simulink library "VIS_LIB"  (Simulink 8.6)
settings: Solver=ode45  StartTime=0.0  StopTime=10.0  RelTol=1e-3
undefined symbols (not defined in the file): AC, SIXOSEM_F_WD_AC_MASTER
libraries: cdsFilt x376, cdsEpicsOut x253, cdsEpicsIn x179, cdsTP x123, VIS_LIB x95, cdsMuxMatrix x91, cdsEpicsStringIn x75, cdsFiltCtrl x72, cdsFunctionCall x70, cdsRms x59, KAGRA_UTIL x25, STATE_BIO_MASTER x5
(part 29 of 38)

== system VIS_LIB/MODAL/inputproc/CAL_GAS ==
  note: #DAQ Channels
      |
      | M1_OUT 256
      | M2_OUT 256
      | M3_OUT 256
      | M4_OUT 256
      | M5_OUT 256
      | M1_IN1 128
      | M2_IN1 128
      | M3_IN1 128
      | M4_IN1 128
      | M5_IN1 128
  LEN_IN : Inport
  TRA_IN : Inport  Port=2
  VER_IN : Inport  Port=3
  ROL_IN : Inport  Port=4
  PIT_IN : Inport  Port=5
  M1 : cdsFilt/Subsystem  Tag=cdsFilt  Description=|
      | Purpose:                                                                                                                                                                                                                                  
      | Standard CDS IIR filter module.                                                                                                                                                                                                           
      |                                                                                                                                                                                                                                           
      | Operation:                                                                                                                                                                                                                                
      | Consists of 10 second order section IIR filters, plus a ramped gain stage. In FE code, also provides pre-defined test points and excitation channel inputs. The filter coefficients are defined in the LIGO system using the 'foton' tool.
      |                                                                                                                                                                                                                                           
      | Usage:                                                                                                                                                                                                                                    
      | Name the part with the desired filter module name.
      settings: AttributesFormatString=%<Tag>
  M2 : cdsFilt/Subsystem  Tag=cdsFilt  Description=|
      | Purpose:                                                                                                                                                                                                                                  
      | Standard CDS IIR filter module.                                                                                                                                                                                                           
      |                                                                                                                                                                                                                                           
      | Operation:                                                                                                                                                                                                                                
      | Consists of 10 second order section IIR filters, plus a ramped gain stage. In FE code, also provides pre-defined test points and excitation channel inputs. The filter coefficients are defined in the LIGO system using the 'foton' tool.
      |                                                                                                                                                                                                                                           
      | Usage:                                                                                                                                                                                                                                    
      | Name the part with the desired filter module name.
      settings: AttributesFormatString=%<Tag>
  M3 : cdsFilt/Subsystem  Tag=cdsFilt  Description=|
      | Purpose:                                                                                                                                                                                                                                  
      | Standard CDS IIR filter module.                                                                                                                                                                                                           
      |                                                                                                                                                                                                                                           
      | Operation:                                                                                                                                                                                                                                
      | Consists of 10 second order section IIR filters, plus a ramped gain stage. In FE code, also provides pre-defined test points and excitation channel inputs. The filter coefficients are defined in the LIGO system using the 'foton' tool.
      |                                                                                                                                                                                                                                           
      | Usage:                                                                                                                                                                                                                                    
      | Name the part with the desired filter module name.
      settings: AttributesFormatString=%<Tag>
  M4 : cdsFilt/Subsystem  Tag=cdsFilt  Description=|
      | Purpose:                                                                                                                                                                                                                                  
      | Standard CDS IIR filter module.                                                                                                                                                                                                           
      |                                                                                                                                                                                                                                           
      | Operation:                                                                                                                                                                                                                                
      | Consists of 10 second order section IIR filters, plus a ramped gain stage. In FE code, also provides pre-defined test points and excitation channel inputs. The filter coefficients are defined in the LIGO system using the 'foton' tool.
      |                                                                                                                                                                                                                                           
      | Usage:                                                                                                                                                                                                                                    
      | Name the part with the desired filter module name.
      settings: AttributesFormatString=%<Tag>
  M5 : cdsFilt/Subsystem  Tag=cdsFilt  Description=|
      | Purpose:                                                                                                                                                                                                                                  
      | Standard CDS IIR filter module.                                                                                                                                                                                                           
      |                                                                                                                                                                                                                                           
      | Operation:                                                                                                                                                                                                                                
      | Consists of 10 second order section IIR filters, plus a ramped gain stage. In FE code, also provides pre-defined test points and excitation channel inputs. The filter coefficients are defined in the LIGO system using the 'foton' tool.
      |                                                                                                                                                                                                                                           
      | Usage:                                                                                                                                                                                                                                    
      | Name the part with the desired filter module name.
      settings: AttributesFormatString=%<Tag>
  LEN_OUT : Outport
  TRA_OUT : Outport  Port=2
  VER_OUT : Outport  Port=3
  ROL_OUT : Outport  Port=4
  PIT_OUT : Outport  Port=5
  wires:
  M1/1 -> LEN_OUT/1
  LEN_IN/1 -> M1/1
  M5/1 -> PIT_OUT/1
  PIT_IN/1 -> M5/1
  ROL_IN/1 -> M4/1
  M4/1 -> ROL_OUT/1
  M2/1 -> TRA_OUT/1
  TRA_IN/1 -> M2/1
  VER_IN/1 -> M3/1
  M3/1 -> VER_OUT/1

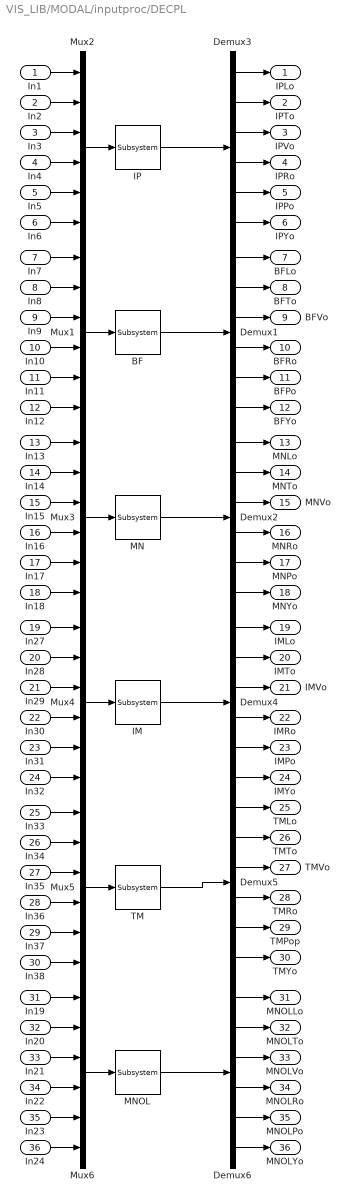
== system VIS_LIB/MODAL/inputproc/DECPL ==
  In1 : Inport
  In2 : Inport  Port=2
  In3 : Inport  Port=3
  In4 : Inport  Port=4
  In5 : Inport  Port=5
  In6 : Inport  Port=6
  In7 : Inport  Port=7
  In8 : Inport  Port=8
  In9 : Inport  Port=9
  In10 : Inport  Port=10
  In11 : Inport  Port=11
  In12 : Inport  Port=12
  In13 : Inport  Port=13
  In14 : Inport  Port=14
  In15 : Inport  Port=15
  In16 : Inport  Port=16
  In17 : Inport  Port=17
  In18 : Inport  Port=18
  In27 : Inport  Port=19
  In28 : Inport  Port=20
  In29 : Inport  Port=21
  In30 : Inport  Port=22
  In31 : Inport  Port=23
  In32 : Inport  Port=24
  In33 : Inport  Port=25
  In34 : Inport  Port=26
  In35 : Inport  Port=27
  In36 : Inport  Port=28
  In37 : Inport  Port=29
  In38 : Inport  Port=30
  In19 : Inport  Port=31
  In20 : Inport  Port=32
  In21 : Inport  Port=33
  In22 : Inport  Port=34
  In23 : Inport  Port=35
  In24 : Inport  Port=36
  BF : cdsMuxMatrix/Subsystem  Tag=cdsMuxMatrix  Description=Any size matrix. Inputs and outputs must be connected using Mux and Demux parts.
      settings: AttributesFormatString=%<Tag>
  Demux{1..6} (6 alike) : Demux  Outputs=6
  IM : cdsMuxMatrix/Subsystem  Tag=cdsMuxMatrix  Description=Any size matrix. Inputs and outputs must be connected using Mux and Demux parts.
      settings: AttributesFormatString=%<Tag>
  IP : cdsMuxMatrix/Subsystem  Tag=cdsMuxMatrix  Description=Any size matrix. Inputs and outputs must be connected using Mux and Demux parts.
      settings: AttributesFormatString=%<Tag>
  MN : cdsMuxMatrix/Subsystem  Tag=cdsMuxMatrix  Description=Any size matrix. Inputs and outputs must be connected using Mux and Demux parts.
      settings: AttributesFormatString=%<Tag>
  MNOL : cdsMuxMatrix/Subsystem  Tag=cdsMuxMatrix  Description=Any size matrix. Inputs and outputs must be connected using Mux and Demux parts.
      settings: AttributesFormatString=%<Tag>
  Mux{1..6} (6 alike) : Mux  Inputs=6
  TM : cdsMuxMatrix/Subsystem  Tag=cdsMuxMatrix  Description=Any size matrix. Inputs and outputs must be connected using Mux and Demux parts.
      settings: AttributesFormatString=%<Tag>
  IPLo : Outport
  IPTo : Outport  Port=2
  IPVo : Outport  Port=3
  IPRo : Outport  Port=4
  IPPo : Outport  Port=5
  IPYo : Outport  Port=6
  BFLo : Outport  Port=7
  BFTo : Outport  Port=8
  BFVo : Outport  Port=9
  BFRo : Outport  Port=10
  BFPo : Outport  Port=11
  BFYo : Outport  Port=12
  MNLo : Outport  Port=13
  MNTo : Outport  Port=14
  MNVo : Outport  Port=15
  MNRo : Outport  Port=16
  MNPo : Outport  Port=17
  MNYo : Outport  Port=18
  IMLo : Outport  Port=19
  IMTo : Outport  Port=20
  IMVo : Outport  Port=21
  IMRo : Outport  Port=22
  IMPo : Outport  Port=23
  IMYo : Outport  Port=24
  TMLo : Outport  Port=25
  TMTo : Outport  Port=26
  TMVo : Outport  Port=27
  TMRo : Outport  Port=28
  TMPop : Outport  Port=29
  TMYo : Outport  Port=30
  MNOLLo : Outport  Port=31
  MNOLTo : Outport  Port=32
  MNOLVo : Outport  Port=33
  MNOLRo : Outport  Port=34
  MNOLPo : Outport  Port=35
  MNOLYo : Outport  Port=36
  wires:
  In6/1 -> Mux2/6
  Mux2/1 -> IP/1
  In3/1 -> Mux2/3
  In1/1 -> Mux2/1
  IP/1 -> Demux3/1
  In5/1 -> Mux2/5
  In2/1 -> Mux2/2
  In4/1 -> Mux2/4
  In12/1 -> Mux1/6
  Mux1/1 -> BF/1
  In9/1 -> Mux1/3
  In7/1 -> Mux1/1
  BF/1 -> Demux1/1
  In11/1 -> Mux1/5
  In8/1 -> Mux1/2
  In10/1 -> Mux1/4
  In18/1 -> Mux3/6
  Mux3/1 -> MN/1
  In15/1 -> Mux3/3
  In13/1 -> Mux3/1
  MN/1 -> Demux2/1
  In17/1 -> Mux3/5
  In14/1 -> Mux3/2
  In16/1 -> Mux3/4
  Mux4/1 -> IM/1
  IM/1 -> Demux4/1
  In30/1 -> Mux4/4
  In27/1 -> Mux4/1
  In29/1 -> Mux4/3
  In28/1 -> Mux4/2
  In32/1 -> Mux4/6
  In31/1 -> Mux4/5
  In38/1 -> Mux5/6
  Mux5/1 -> TM/1
  In35/1 -> Mux5/3
  In33/1 -> Mux5/1
  TM/1 -> Demux5/1
  In37/1 -> Mux5/5
  In34/1 -> Mux5/2
  In36/1 -> Mux5/4
  Demux3/6 -> IPYo/1
  Demux1/1 -> BFLo/1
  Demux1/2 -> BFTo/1
  Demux1/3 -> BFVo/1
  Demux1/4 -> BFRo/1
  Demux1/5 -> BFPo/1
  Demux1/6 -> BFYo/1
  Demux2/1 -> MNLo/1
  Demux2/2 -> MNTo/1
  Demux2/3 -> MNVo/1
  Demux2/4 -> MNRo/1
  Demux2/5 -> MNPo/1
  Demux2/6 -> MNYo/1
  Demux4/1 -> IMLo/1
  Demux4/2 -> IMTo/1
  Demux4/3 -> IMVo/1
  Demux4/4 -> IMRo/1
  Demux4/5 -> IMPo/1
  Demux4/6 -> IMYo/1
  Demux5/1 -> TMLo/1
  Demux3/1 -> IPLo/1
  Demux3/2 -> IPTo/1
  Demux3/3 -> IPVo/1
  Demux3/4 -> IPRo/1
  Demux3/5 -> IPPo/1
  Demux5/2 -> TMTo/1
  Demux5/3 -> TMVo/1
  Demux5/4 -> TMRo/1
  Demux5/5 -> TMPop/1
  Demux5/6 -> TMYo/1
  In24/1 -> Mux6/6
  Mux6/1 -> MNOL/1
  In21/1 -> Mux6/3
  In19/1 -> Mux6/1
  MNOL/1 -> Demux6/1
  In23/1 -> Mux6/5
  In20/1 -> Mux6/2
  In22/1 -> Mux6/4
  Demux6/2 -> MNOLTo/1
  Demux6/3 -> MNOLVo/1
  Demux6/4 -> MNOLRo/1
  Demux6/5 -> MNOLPo/1
  Demux6/6 -> MNOLYo/1
  Demux6/1 -> MNOLLo/1

== system VIS_LIB/MODAL/inputproc/EUL ==
  In1 : Inport
  In2 : Inport  Port=2
  In3 : Inport  Port=3
  In4 : Inport  Port=4
  In5 : Inport  Port=5
  In6 : Inport  Port=6
  In7 : Inport  Port=7
  In8 : Inport  Port=8
  In9 : Inport  Port=9
  In10 : Inport  Port=10
  In11 : Inport  Port=11
  In12 : Inport  Port=12
  In13 : Inport  Port=13
  In14 : Inport  Port=14
  In15 : Inport  Port=15
  In16 : Inport  Port=16
  In17 : Inport  Port=17
  In18 : Inport  Port=18
  In19 : Inport  Port=19
  In20 : Inport  Port=20
  In21 : Inport  Port=21
  In22 : Inport  Port=22
  In23 : Inport  Port=23
  In24 : Inport  Port=24
  In25 : Inport  Port=25
  In26 : Inport  Port=26
  In27 : Inport  Port=27
  In28 : Inport  Port=28
  In29 : Inport  Port=29
  In30 : Inport  Port=30
  In31 : Inport  Port=31
  In32 : Inport  Port=32
  In33 : Inport  Port=33
  In34 : Inport  Port=34
  In35 : Inport  Port=35
  In36 : Inport  Port=36
  BF : VIS_LIB/UTILs/FBs_6DOF_DQ
  IM : VIS_LIB/UTILs/FBs_6DOF_DQ
  IP : VIS_LIB/UTILs/FBs_6DOF_DQ
  MN : VIS_LIB/UTILs/FBs_6DOF_DQ
  MNOL : VIS_LIB/UTILs/FBs_6DOF_DQ
  TM : VIS_LIB/UTILs/FBs_6DOF_DQ
  Out1 : Outport
  Out2 : Outport  Port=2
  Out3 : Outport  Port=3
  Out4 : Outport  Port=4
  Out5 : Outport  Port=5
  Out6 : Outport  Port=6
  Out7 : Outport  Port=7
  Out8 : Outport  Port=8
  Out9 : Outport  Port=9
  Out10 : Outport  Port=10
  Out11 : Outport  Port=11
  Out12 : Outport  Port=12
  Out13 : Outport  Port=13
  Out14 : Outport  Port=14
  Out15 : Outport  Port=15
  Out16 : Outport  Port=16
  Out17 : Outport  Port=17
  Out18 : Outport  Port=18
  Out19 : Outport  Port=19
  Out20 : Outport  Port=20
  Out21 : Outport  Port=21
  Out22 : Outport  Port=22
  Out23 : Outport  Port=23
  Out24 : Outport  Port=24
  Out25 : Outport  Port=25
  Out26 : Outport  Port=26
  Out27 : Outport  Port=27
  Out28 : Outport  Port=28
  Out29 : Outport  Port=29
  Out30 : Outport  Port=30
  Out31 : Outport  Port=31
  Out32 : Outport  Port=32
  Out33 : Outport  Port=33
  Out34 : Outport  Port=34
  Out35 : Outport  Port=35
  Out36 : Outport  Port=36
  wires:
  In16/1 -> MN/4
  In15/1 -> MN/3
  In14/1 -> MN/2
  In12/1 -> BF/6
  In13/1 -> MN/1
  In11/1 -> BF/5
  In10/1 -> BF/4
  In9/1 -> BF/3
  In8/1 -> BF/2
  TM/5 -> Out29/1
  TM/2 -> Out26/1
  TM/3 -> Out27/1
  In30/1 -> TM/6
  TM/1 -> Out25/1
  In23/1 -> IM/5
  In22/1 -> IM/4
  In21/1 -> IM/3
  In20/1 -> IM/2
  BF/6 -> Out12/1
  In19/1 -> IM/1
  MN/2 -> Out14/1
  MN/1 -> Out13/1
  In17/1 -> MN/5
  In18/1 -> MN/6
  IM/2 -> Out20/1
  MN/3 -> Out15/1
  IM/1 -> Out19/1
  In24/1 -> IM/6
  TM/4 -> Out28/1
  BF/1 -> Out7/1
  MN/6 -> Out18/1
  MN/5 -> Out17/1
  MN/4 -> Out16/1
  TM/6 -> Out30/1
  In7/1 -> BF/1
  In6/1 -> IP/6
  In5/1 -> IP/5
  In3/1 -> IP/3
  In4/1 -> IP/4
  In29/1 -> TM/5
  In28/1 -> TM/4
  In27/1 -> TM/3
  In26/1 -> TM/2
  BF/5 -> Out11/1
  BF/4 -> Out10/1
  BF/3 -> Out9/1
  BF/2 -> Out8/1
  IP/3 -> Out3/1
  IP/2 -> Out2/1
  IP/1 -> Out1/1
  In1/1 -> IP/1
  In25/1 -> TM/1
  IM/6 -> Out24/1
  IM/5 -> Out23/1
  IM/3 -> Out21/1
  IM/4 -> Out22/1
  In2/1 -> IP/2
  IP/6 -> Out6/1
  IP/5 -> Out5/1
  IP/4 -> Out4/1
  MNOL/5 -> Out35/1
  MNOL/2 -> Out32/1
  MNOL/3 -> Out33/1
  In36/1 -> MNOL/6
  MNOL/4 -> Out34/1
  MNOL/6 -> Out36/1
  In35/1 -> MNOL/5
  In34/1 -> MNOL/4
  In33/1 -> MNOL/3
  In32/1 -> MNOL/2
  In31/1 -> MNOL/1
  MNOL/1 -> Out31/1

== system VIS_LIB/MODAL/inputproc/OL_PROC ==
  MNSEG1 : Inport
  MNSEG2 : Inport  Port=2
  MNSEG3 : Inport  Port=3
  MNSEG4 : Inport  Port=4
  TILT_SEG1 : Inport  Port=5
  TILT_SEG2 : Inport  Port=6
  TILT_SEG3 : Inport  Port=7
  TILT_SEG4 : Inport  Port=8
  LEN_SEG1 : Inport  Port=9
  LEN_SEG2 : Inport  Port=10
  LEN_SEG3 : Inport  Port=11
  LEN_SEG4 : Inport  Port=12
  MN_TILT : Subsystem
  TM_LEN : Subsystem
  TM_TILT : Subsystem
  MNV : Outport
  MNH : Outport  Port=2
  TMV1 : Outport  Port=3
  TMV2 : Outport  Port=4
  TMH1 : Outport  Port=5
  TMH2 : Outport  Port=6
  wires:
  MNSEG2/1 -> MN_TILT/2(SEG2_in)
  MNSEG1/1 -> MN_TILT/1(SEG1_in)
  MNSEG4/1 -> MN_TILT/4(SEG4_in)
  MN_TILT/1(V) -> MNV/1
  MN_TILT/2(H) -> MNH/1
  MNSEG3/1 -> MN_TILT/3(SEG3_in)
  TILT_SEG1/1 -> TM_TILT/1(SEG1_in)
  TILT_SEG2/1 -> TM_TILT/2(SEG2_in)
  TILT_SEG4/1 -> TM_TILT/4(SEG4_in)
  TILT_SEG3/1 -> TM_TILT/3(SEG3_in)
  LEN_SEG1/1 -> TM_LEN/1(SEG1_in)
  LEN_SEG2/1 -> TM_LEN/2(SEG2_in)
  LEN_SEG3/1 -> TM_LEN/3(SEG3_in)
  LEN_SEG4/1 -> TM_LEN/4(SEG4_in)
  TM_TILT/1(V) -> TMV1/1
  TM_TILT/2(H) -> TMH1/1
  TM_LEN/1(V) -> TMV2/1
  TM_LEN/2(H) -> TMH2/1

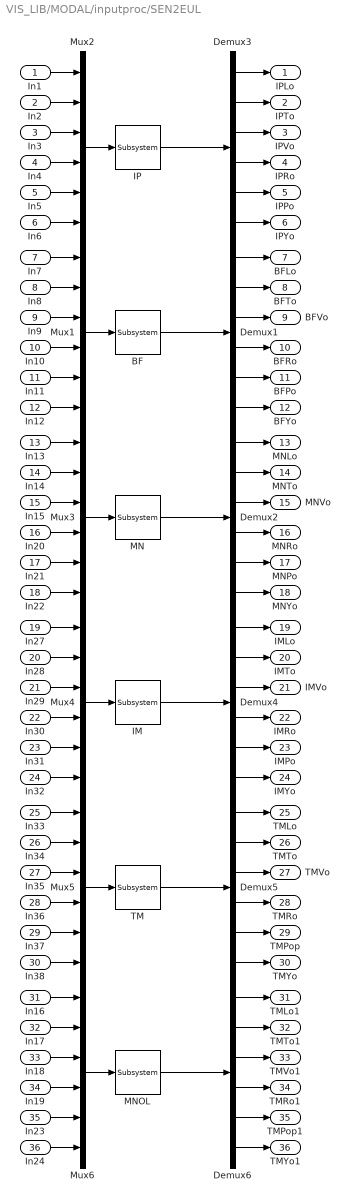
== system VIS_LIB/MODAL/inputproc/SEN2EUL ==
  In1 : Inport
  In2 : Inport  Port=2
  In3 : Inport  Port=3
  In4 : Inport  Port=4
  In5 : Inport  Port=5
  In6 : Inport  Port=6
  In7 : Inport  Port=7
  In8 : Inport  Port=8
  In9 : Inport  Port=9
  In10 : Inport  Port=10
  In11 : Inport  Port=11
  In12 : Inport  Port=12
  In13 : Inport  Port=13
  In14 : Inport  Port=14
  In15 : Inport  Port=15
  In20 : Inport  Port=16
  In21 : Inport  Port=17
  In22 : Inport  Port=18
  In27 : Inport  Port=19
  In28 : Inport  Port=20
  In29 : Inport  Port=21
  In30 : Inport  Port=22
  In31 : Inport  Port=23
  In32 : Inport  Port=24
  In33 : Inport  Port=25
  In34 : Inport  Port=26
  In35 : Inport  Port=27
  In36 : Inport  Port=28
  In37 : Inport  Port=29
  In38 : Inport  Port=30
  In16 : Inport  Port=31
  In17 : Inport  Port=32
  In18 : Inport  Port=33
  In19 : Inport  Port=34
  In23 : Inport  Port=35
  In24 : Inport  Port=36
  BF : cdsMuxMatrix/Subsystem  Tag=cdsMuxMatrix  Description=Any size matrix. Inputs and outputs must be connected using Mux and Demux parts.
      settings: AttributesFormatString=%<Tag>
  Demux{1..6} (6 alike) : Demux  Outputs=6
  IM : cdsMuxMatrix/Subsystem  Tag=cdsMuxMatrix  Description=Any size matrix. Inputs and outputs must be connected using Mux and Demux parts.
      settings: AttributesFormatString=%<Tag>
  IP : cdsMuxMatrix/Subsystem  Tag=cdsMuxMatrix  Description=Any size matrix. Inputs and outputs must be connected using Mux and Demux parts.
      settings: AttributesFormatString=%<Tag>
  MN : cdsMuxMatrix/Subsystem  Tag=cdsMuxMatrix  Description=Any size matrix. Inputs and outputs must be connected using Mux and Demux parts.
      settings: AttributesFormatString=%<Tag>
  MNOL : cdsMuxMatrix/Subsystem  Tag=cdsMuxMatrix  Description=Any size matrix. Inputs and outputs must be connected using Mux and Demux parts.
      settings: AttributesFormatString=%<Tag>
  Mux{1..6} (6 alike) : Mux  Inputs=6
  TM : cdsMuxMatrix/Subsystem  Tag=cdsMuxMatrix  Description=Any size matrix. Inputs and outputs must be connected using Mux and Demux parts.
      settings: AttributesFormatString=%<Tag>
  IPLo : Outport
  IPTo : Outport  Port=2
  IPVo : Outport  Port=3
  IPRo : Outport  Port=4
  IPPo : Outport  Port=5
  IPYo : Outport  Port=6
  BFLo : Outport  Port=7
  BFTo : Outport  Port=8
  BFVo : Outport  Port=9
  BFRo : Outport  Port=10
  BFPo : Outport  Port=11
  BFYo : Outport  Port=12
  MNLo : Outport  Port=13
  MNTo : Outport  Port=14
  MNVo : Outport  Port=15
  MNRo : Outport  Port=16
  MNPo : Outport  Port=17
  MNYo : Outport  Port=18
  IMLo : Outport  Port=19
  IMTo : Outport  Port=20
  IMVo : Outport  Port=21
  IMRo : Outport  Port=22
  IMPo : Outport  Port=23
  IMYo : Outport  Port=24
  TMLo : Outport  Port=25
  TMTo : Outport  Port=26
  TMVo : Outport  Port=27
  TMRo : Outport  Port=28
  TMPop : Outport  Port=29
  TMYo : Outport  Port=30
  TMLo1 : Outport  Port=31
  TMTo1 : Outport  Port=32
  TMVo1 : Outport  Port=33
  TMRo1 : Outport  Port=34
  TMPop1 : Outport  Port=35
  TMYo1 : Outport  Port=36
  wires:
  In6/1 -> Mux2/6
  Mux2/1 -> IP/1
  In3/1 -> Mux2/3
  In1/1 -> Mux2/1
  IP/1 -> Demux3/1
  In5/1 -> Mux2/5
  In2/1 -> Mux2/2
  In4/1 -> Mux2/4
  In12/1 -> Mux1/6
  Mux1/1 -> BF/1
  In9/1 -> Mux1/3
  In7/1 -> Mux1/1
  BF/1 -> Demux1/1
  In11/1 -> Mux1/5
  In8/1 -> Mux1/2
  In10/1 -> Mux1/4
  Mux3/1 -> MN/1
  In15/1 -> Mux3/3
  In13/1 -> Mux3/1
  MN/1 -> Demux2/1
  In14/1 -> Mux3/2
  Mux4/1 -> IM/1
  IM/1 -> Demux4/1
  In21/1 -> Mux3/5
  In20/1 -> Mux3/4
  In22/1 -> Mux3/6
  In30/1 -> Mux4/4
  In27/1 -> Mux4/1
  In29/1 -> Mux4/3
  In28/1 -> Mux4/2
  In32/1 -> Mux4/6
  In31/1 -> Mux4/5
  In38/1 -> Mux5/6
  Mux5/1 -> TM/1
  In35/1 -> Mux5/3
  In33/1 -> Mux5/1
  TM/1 -> Demux5/1
  In37/1 -> Mux5/5
  In34/1 -> Mux5/2
  In36/1 -> Mux5/4
  Demux3/6 -> IPYo/1
  Demux1/1 -> BFLo/1
  Demux1/2 -> BFTo/1
  Demux1/3 -> BFVo/1
  Demux1/4 -> BFRo/1
  Demux1/5 -> BFPo/1
  Demux1/6 -> BFYo/1
  Demux2/1 -> MNLo/1
  Demux2/2 -> MNTo/1
  Demux2/3 -> MNVo/1
  Demux2/4 -> MNRo/1
  Demux2/5 -> MNPo/1
  Demux2/6 -> MNYo/1
  Demux4/1 -> IMLo/1
  Demux4/2 -> IMTo/1
  Demux4/3 -> IMVo/1
  Demux4/4 -> IMRo/1
  Demux4/5 -> IMPo/1
  Demux4/6 -> IMYo/1
  Demux5/1 -> TMLo/1
  Demux3/1 -> IPLo/1
  Demux3/2 -> IPTo/1
  Demux3/3 -> IPVo/1
  Demux3/4 -> IPRo/1
  Demux3/5 -> IPPo/1
  Demux5/2 -> TMTo/1
  Demux5/3 -> TMVo/1
  Demux5/4 -> TMRo/1
  Demux5/5 -> TMPop/1
  Demux5/6 -> TMYo/1
  In24/1 -> Mux6/6
  Mux6/1 -> MNOL/1
  In18/1 -> Mux6/3
  MNOL/1 -> Demux6/1
  In23/1 -> Mux6/5
  In17/1 -> Mux6/2
  In19/1 -> Mux6/4
  Demux6/2 -> TMTo1/1
  Demux6/3 -> TMVo1/1
  Demux6/4 -> TMRo1/1
  Demux6/5 -> TMPop1/1
  Demux6/6 -> TMYo1/1
  Demux6/1 -> TMLo1/1
  In16/1 -> Mux6/1

== system VIS_LIB/MODAL/inputproc/SENSIN ==
  IPLVDT_H1 : Inport
  IPLVDT_H2 : Inport  Port=2
  IPLVDT_H3 : Inport  Port=3
  BFLVDT_V1 : Inport  Port=4
  BFLVDT_V2 : Inport  Port=5
  BFLVDT_V3 : Inport  Port=6
  BFLVDT_H1 : Inport  Port=7
  BFLVDT_H2 : Inport  Port=8
  BFLVDT_H3 : Inport  Port=9
  MCPS_V1 : Inport  Port=10
  MCPS_V2 : Inport  Port=11
  MCPS_V3 : Inport  Port=12
  MCPS_H1 : Inport  Port=13
  MCPS_H2 : Inport  Port=14
  MNPS_H3 : Inport  Port=15
  IMPS_V1 : Inport  Port=16
  IMPS_V2 : Inport  Port=17
  IMPS_V3 : Inport  Port=18
  IMPS_H1 : Inport  Port=19
  IMPS_H2 : Inport  Port=20
  IMPS_H3 : Inport  Port=21
  MNOL_V : Inport  Port=22
  MNOL_H4 : Inport  Port=23
  TMOLV1 : Inport  Port=24
  TMOLV2 : Inport  Port=25
  TMOLH1 : Inport  Port=26
  TMOLH2 : Inport  Port=27
  BF : VIS_LIB/UTILs/6COILs_DQ
  Ground{1..7,9..10} (9 alike) : Ground
  IM : VIS_LIB/UTILs/6COILs_DQ
  IP : VIS_LIB/UTILs/6COILs_DQ
  MN : VIS_LIB/UTILs/6COILs_DQ
  MNOL : VIS_LIB/UTILs/6COILs_DQ
  TM : VIS_LIB/UTILs/6COILs_DQ
  IPV1 : Outport
  IPV2 : Outport  Port=2
  IPV3 : Outport  Port=3
  IPH1 : Outport  Port=4
  IPH2 : Outport  Port=5
  IPH3 : Outport  Port=6
  BFV1 : Outport  Port=7
  BFV2 : Outport  Port=8
  BFV3 : Outport  Port=9
  BFH1 : Outport  Port=10
  BFH2 : Outport  Port=11
  BFH3 : Outport  Port=12
  MNV1 : Outport  Port=13
  MNV2 : Outport  Port=14
  MNV3 : Outport  Port=15
  MNH1 : Outport  Port=16
  MNH2 : Outport  Port=17
  MNH3 : Outport  Port=18
  IMV1 : Outport  Port=19
  IMV2 : Outport  Port=20
  IMV3 : Outport  Port=21
  IMH1 : Outport  Port=22
  IMH2 : Outport  Port=23
  IMH3 : Outport  Port=24
  IMV4 : Outport  Port=25
  IMV5 : Outport  Port=26
  IMV6 : Outport  Port=27
  IMH4 : Outport  Port=28
  IMH5 : Outport  Port=29
  IMH6 : Outport  Port=30
  MNOLV1 : Outport  Port=31
  MNOLV2 : Outport  Port=32
  MNOLV3 : Outport  Port=33
  MNOLH1 : Outport  Port=34
  MNOLH2 : Outport  Port=35
  MNOLH3 : Outport  Port=36
  wires:
  IPLVDT_H1/1 -> IP/4
  IPLVDT_H2/1 -> IP/5
  IPLVDT_H3/1 -> IP/6
  BFLVDT_V1/1 -> BF/1
  BFLVDT_V2/1 -> BF/2
  BFLVDT_V3/1 -> BF/3
  BFLVDT_H1/1 -> BF/4
  BFLVDT_H2/1 -> BF/5
  BFLVDT_H3/1 -> BF/6
  MCPS_V1/1 -> MN/1
  MCPS_V2/1 -> MN/2
  MCPS_V3/1 -> MN/3
  MCPS_H1/1 -> MN/4
  MCPS_H2/1 -> MN/5
  MNPS_H3/1 -> MN/6
  IMPS_V1/1 -> IM/1
  IMPS_V2/1 -> IM/2
  IMPS_V3/1 -> IM/3
  IMPS_H1/1 -> IM/4
  IMPS_H2/1 -> IM/5
  IMPS_H3/1 -> IM/6
  Ground2/1 -> IP/1
  Ground1/1 -> IP/2
  Ground3/1 -> IP/3
  IP/5 -> IPH2/1
  IP/4 -> IPH1/1
  IP/6 -> IPH3/1
  BF/1 -> BFV1/1
  BF/3 -> BFV3/1
  BF/5 -> BFH2/1
  BF/6 -> BFH3/1
  BF/2 -> BFV2/1
  BF/4 -> BFH1/1
  IM/6 -> IMH3/1
  IM/5 -> IMH2/1
  IM/4 -> IMH1/1
  IM/3 -> IMV3/1
  IM/2 -> IMV2/1
  IM/1 -> IMV1/1
  MN/6 -> MNH3/1
  MN/5 -> MNH2/1
  MN/4 -> MNH1/1
  MN/3 -> MNV3/1
  MN/2 -> MNV2/1
  MN/1 -> MNV1/1
  IP/1 -> IPV1/1
  IP/2 -> IPV2/1
  IP/3 -> IPV3/1
  MNOL_V/1 -> MNOL/1
  MNOL_H4/1 -> MNOL/4
  TMOLV2/1 -> TM/2
  TMOLH1/1 -> TM/4
  TMOLH2/1 -> TM/5
  TM/6 -> IMH6/1
  TM/5 -> IMH5/1
  TM/4 -> IMH4/1
  TM/3 -> IMV6/1
  TM/2 -> IMV5/1
  TMOLV1/1 -> TM/1
  Ground9/1 -> TM/3
  Ground10/1 -> TM/6
  TM/1 -> IMV4/1
  MNOL/6 -> MNOLH3/1
  MNOL/5 -> MNOLH2/1
  MNOL/4 -> MNOLH1/1
  MNOL/3 -> MNOLV3/1
  MNOL/2 -> MNOLV2/1
  Ground5/1 -> MNOL/3
  Ground4/1 -> MNOL/6
  MNOL/1 -> MNOLV1/1
  Ground7/1 -> MNOL/2
  Ground6/1 -> MNOL/5

== system VIS_LIB/MODAL/inputproc/SENSIN_GAS ==
  note: #DAQ Channels
      |
      | F0_OUT 256
      | F1_OUT 256
      | F2_OUT 256
      | F3_OUT 256
      | BF_OUT 256
  iF0 : Inport
  iF1 : Inport  Port=2
  iF2 : Inport  Port=3
  iF3 : Inport  Port=4
  iBF : Inport  Port=5
  BF : cdsFilt/Subsystem  Tag=cdsFilt  Description=|
      | Purpose:                                                                                                                                                                                                                                  
      | Standard CDS IIR filter module.                                                                                                                                                                                                           
      |                                                                                                                                                                                                                                           
      | Operation:                                                                                                                                                                                                                                
      | Consists of 10 second order section IIR filters, plus a ramped gain stage. In FE code, also provides pre-defined test points and excitation channel inputs. The filter coefficients are defined in the LIGO system using the 'foton' tool.
      |                                                                                                                                                                                                                                           
      | Usage:                                                                                                                                                                                                                                    
      | Name the part with the desired filter module name.
      settings: AttributesFormatString=%<Tag>
  F0 : cdsFilt/Subsystem  Tag=cdsFilt  Description=|
      | Purpose:                                                                                                                                                                                                                                  
      | Standard CDS IIR filter module.                                                                                                                                                                                                           
      |                                                                                                                                                                                                                                           
      | Operation:                                                                                                                                                                                                                                
      | Consists of 10 second order section IIR filters, plus a ramped gain stage. In FE code, also provides pre-defined test points and excitation channel inputs. The filter coefficients are defined in the LIGO system using the 'foton' tool.
      |                                                                                                                                                                                                                                           
      | Usage:                                                                                                                                                                                                                                    
      | Name the part with the desired filter module name.
      settings: AttributesFormatString=%<Tag>
  F1 : cdsFilt/Subsystem  Tag=cdsFilt  Description=|
      | Purpose:                                                                                                                                                                                                                                  
      | Standard CDS IIR filter module.                                                                                                                                                                                                           
      |                                                                                                                                                                                                                                           
      | Operation:                                                                                                                                                                                                                                
      | Consists of 10 second order section IIR filters, plus a ramped gain stage. In FE code, also provides pre-defined test points and excitation channel inputs. The filter coefficients are defined in the LIGO system using the 'foton' tool.
      |                                                                                                                                                                                                                                           
      | Usage:                                                                                                                                                                                                                                    
      | Name the part with the desired filter module name.
      settings: AttributesFormatString=%<Tag>
  F2 : cdsFilt/Subsystem  Tag=cdsFilt  Description=|
      | Purpose:                                                                                                                                                                                                                                  
      | Standard CDS IIR filter module.                                                                                                                                                                                                           
      |                                                                                                                                                                                                                                           
      | Operation:                                                                                                                                                                                                                                
      | Consists of 10 second order section IIR filters, plus a ramped gain stage. In FE code, also provides pre-defined test points and excitation channel inputs. The filter coefficients are defined in the LIGO system using the 'foton' tool.
      |                                                                                                                                                                                                                                           
      | Usage:                                                                                                                                                                                                                                    
      | Name the part with the desired filter module name.
      settings: AttributesFormatString=%<Tag>
  F3 : cdsFilt/Subsystem  Tag=cdsFilt  Description=|
      | Purpose:                                                                                                                                                                                                                                  
      | Standard CDS IIR filter module.                                                                                                                                                                                                           
      |                                                                                                                                                                                                                                           
      | Operation:                                                                                                                                                                                                                                
      | Consists of 10 second order section IIR filters, plus a ramped gain stage. In FE code, also provides pre-defined test points and excitation channel inputs. The filter coefficients are defined in the LIGO system using the 'foton' tool.
      |                                                                                                                                                                                                                                           
      | Usage:                                                                                                                                                                                                                                    
      | Name the part with the desired filter module name.
      settings: AttributesFormatString=%<Tag>
  oF0 : Outport
  oF1 : Outport  Port=2
  oF2 : Outport  Port=3
  oF3 : Outport  Port=4
  oBF : Outport  Port=5
  wires:
  BF/1 -> oBF/1
  iBF/1 -> BF/1
  F3/1 -> oF3/1
  iF3/1 -> F3/1
  F2/1 -> oF2/1
  iF2/1 -> F2/1
  F1/1 -> oF1/1
  iF1/1 -> F1/1
  F0/1 -> oF0/1
  iF0/1 -> F0/1

== system VIS_LIB/MODAL/inputproc_forQUA/CAL ==
  In1 : Inport
  In2 : Inport  Port=2
  In3 : Inport  Port=3
  In4 : Inport  Port=4
  In5 : Inport  Port=5
  In6 : Inport  Port=6
  In7 : Inport  Port=7
  In8 : Inport  Port=8
  In9 : Inport  Port=9
  In10 : Inport  Port=10
  In11 : Inport  Port=11
  In12 : Inport  Port=12
  In13 : Inport  Port=13
  In14 : Inport  Port=14
  In15 : Inport  Port=15
  In16 : Inport  Port=16
  In17 : Inport  Port=17
  In18 : Inport  Port=18
  In19 : Inport  Port=19
  In20 : Inport  Port=20
  In21 : Inport  Port=21
  In22 : Inport  Port=22
  In23 : Inport  Port=23
  In24 : Inport  Port=24
  In25 : Inport  Port=25
  In26 : Inport  Port=26
  In27 : Inport  Port=27
  In28 : Inport  Port=28
  In29 : Inport  Port=29
  In30 : Inport  Port=30
  In31 : Inport  Port=31
  In32 : Inport  Port=32
  In33 : Inport  Port=33
  In34 : Inport  Port=34
  In35 : Inport  Port=35
  In36 : Inport  Port=36
  In37 : Inport  Port=37
  In38 : Inport  Port=38
  In39 : Inport  Port=39
  In40 : Inport  Port=40
  In41 : Inport  Port=41
  BF : Subsystem
  GAS : Subsystem
  IM : Subsystem
  IP : Subsystem
  MN : Subsystem
  MNOL : Subsystem
  TM : Subsystem
  Out1 : Outport
  Out2 : Outport  Port=2
  Out3 : Outport  Port=3
  Out4 : Outport  Port=4
  Out5 : Outport  Port=5
  Out6 : Outport  Port=6
  Out7 : Outport  Port=7
  Out8 : Outport  Port=8
  Out9 : Outport  Port=9
  Out10 : Outport  Port=10
  Out11 : Outport  Port=11
  Out12 : Outport  Port=12
  Out13 : Outport  Port=13
  Out14 : Outport  Port=14
  Out15 : Outport  Port=15
  Out16 : Outport  Port=16
  Out17 : Outport  Port=17
  Out18 : Outport  Port=18
  Out19 : Outport  Port=19
  Out20 : Outport  Port=20
  Out21 : Outport  Port=21
  Out22 : Outport  Port=22
  Out23 : Outport  Port=23
  Out24 : Outport  Port=24
  Out25 : Outport  Port=25
  Out26 : Outport  Port=26
  Out27 : Outport  Port=27
  Out28 : Outport  Port=28
  Out29 : Outport  Port=29
  Out30 : Outport  Port=30
  Out31 : Outport  Port=31
  Out32 : Outport  Port=32
  Out33 : Outport  Port=33
  Out34 : Outport  Port=34
  Out35 : Outport  Port=35
  Out36 : Outport  Port=36
  Out37 : Outport  Port=37
  Out38 : Outport  Port=38
  Out39 : Outport  Port=39
  Out40 : Outport  Port=40
  Out41 : Outport  Port=41
  wires:
  IP/4(ROL_OUT) -> Out4/1
  IP/5(PIT_OUT) -> Out5/1
  IP/6(YAW_OUT) -> Out6/1
  In2/1 -> IP/2(TRA_IN)
  IM/4(ROL_OUT) -> Out22/1
  IM/3(VER_OUT) -> Out21/1
  IM/5(PIT_OUT) -> Out23/1
  IM/6(YAW_OUT) -> Out24/1
  In25/1 -> TM/1(LEN_IN)
  In1/1 -> IP/1(LEN_IN)
  IP/1(LEN_OUT) -> Out1/1
  IP/2(TRA_OUT) -> Out2/1
  IP/3(VER_OUT) -> Out3/1
  BF/2(TRA_OUT) -> Out8/1
  BF/3(VER_OUT) -> Out9/1
  BF/4(ROL_OUT) -> Out10/1
  BF/5(PIT_OUT) -> Out11/1
  In26/1 -> TM/2(TRA_IN)
  In27/1 -> TM/3(VER_IN)
  In28/1 -> TM/4(ROL_IN)
  In29/1 -> TM/5(PIT_IN)
  In4/1 -> IP/4(ROL_IN)
  In3/1 -> IP/3(VER_IN)
  In5/1 -> IP/5(PIT_IN)
  In6/1 -> IP/6(YAW_IN)
  In7/1 -> BF/1(LEN_IN)
  TM/6(YAW_OUT) -> Out30/1
  MN/4(ROL_OUT) -> Out16/1
  MN/5(PIT_OUT) -> Out17/1
  MN/6(YAW_OUT) -> Out18/1
  BF/1(LEN_OUT) -> Out7/1
  TM/4(ROL_OUT) -> Out28/1
  In24/1 -> IM/6(YAW_IN)
  IM/1(LEN_OUT) -> Out19/1
  MN/3(VER_OUT) -> Out15/1
  IM/2(TRA_OUT) -> Out20/1
  In18/1 -> MN/6(YAW_IN)
  In17/1 -> MN/5(PIT_IN)
  MN/1(LEN_OUT) -> Out13/1
  MN/2(TRA_OUT) -> Out14/1
  In19/1 -> IM/1(LEN_IN)
  BF/6(YAW_OUT) -> Out12/1
  In20/1 -> IM/2(TRA_IN)
  In21/1 -> IM/3(VER_IN)
  In22/1 -> IM/4(ROL_IN)
  In23/1 -> IM/5(PIT_IN)
  TM/1(LEN_OUT) -> Out25/1
  In30/1 -> TM/6(YAW_IN)
  TM/3(VER_OUT) -> Out27/1
  TM/2(TRA_OUT) -> Out26/1
  TM/5(PIT_OUT) -> Out29/1
  In8/1 -> BF/2(TRA_IN)
  In9/1 -> BF/3(VER_IN)
  In10/1 -> BF/4(ROL_IN)
  In11/1 -> BF/5(PIT_IN)
  In13/1 -> MN/1(LEN_IN)
  In12/1 -> BF/6(YAW_IN)
  In14/1 -> MN/2(TRA_IN)
  In15/1 -> MN/3(VER_IN)
  In16/1 -> MN/4(ROL_IN)
  In32/1 -> MNOL/2(TRA_IN)
  In33/1 -> MNOL/3(VER_IN)
  In34/1 -> MNOL/4(ROL_IN)
  In35/1 -> MNOL/5(PIT_IN)
  MNOL/6(YAW_OUT) -> Out36/1
  MNOL/4(ROL_OUT) -> Out34/1
  In36/1 -> MNOL/6(YAW_IN)
  MNOL/3(VER_OUT) -> Out33/1
  MNOL/2(TRA_OUT) -> Out32/1
  MNOL/5(PIT_OUT) -> Out35/1
  MNOL/1(LEN_OUT) -> Out31/1
  In31/1 -> MNOL/1(LEN_IN)
  In38/1 -> GAS/2(TRA_IN)
  In39/1 -> GAS/3(VER_IN)
  In40/1 -> GAS/4(ROL_IN)
  In41/1 -> GAS/5(PIT_IN)
  In37/1 -> GAS/1(LEN_IN)
  GAS/5(PIT_OUT) -> Out41/1
  GAS/3(VER_OUT) -> Out39/1
  GAS/2(TRA_OUT) -> Out38/1
  GAS/1(LEN_OUT) -> Out37/1
  GAS/4(ROL_OUT) -> Out40/1

== system VIS_LIB/MODAL/inputproc_forQUA/DECPL ==
  In1 : Inport
  In2 : Inport  Port=2
  In3 : Inport  Port=3
  In4 : Inport  Port=4
  In5 : Inport  Port=5
  In6 : Inport  Port=6
  In7 : Inport  Port=7
  In8 : Inport  Port=8
  In9 : Inport  Port=9
  In10 : Inport  Port=10
  In11 : Inport  Port=11
  In12 : Inport  Port=12
  In13 : Inport  Port=13
  In14 : Inport  Port=14
  In15 : Inport  Port=15
  In16 : Inport  Port=16
  In17 : Inport  Port=17
  In18 : Inport  Port=18
  In27 : Inport  Port=19
  In28 : Inport  Port=20
  In29 : Inport  Port=21
  In30 : Inport  Port=22
  In31 : Inport  Port=23
  In32 : Inport  Port=24
  In33 : Inport  Port=25
  In34 : Inport  Port=26
  In35 : Inport  Port=27
  In36 : Inport  Port=28
  In37 : Inport  Port=29
  In38 : Inport  Port=30
  In19 : Inport  Port=31
  In20 : Inport  Port=32
  In21 : Inport  Port=33
  In22 : Inport  Port=34
  In23 : Inport  Port=35
  In24 : Inport  Port=36
  BF : cdsMuxMatrix/Subsystem  Tag=cdsMuxMatrix  Description=Any size matrix. Inputs and outputs must be connected using Mux and Demux parts.
      settings: AttributesFormatString=%<Tag>
  Demux{1..6} (6 alike) : Demux  Outputs=6
  IM : cdsMuxMatrix/Subsystem  Tag=cdsMuxMatrix  Description=Any size matrix. Inputs and outputs must be connected using Mux and Demux parts.
      settings: AttributesFormatString=%<Tag>
  IP : cdsMuxMatrix/Subsystem  Tag=cdsMuxMatrix  Description=Any size matrix. Inputs and outputs must be connected using Mux and Demux parts.
      settings: AttributesFormatString=%<Tag>
  MN : cdsMuxMatrix/Subsystem  Tag=cdsMuxMatrix  Description=Any size matrix. Inputs and outputs must be connected using Mux and Demux parts.
      settings: AttributesFormatString=%<Tag>
  MNOL : cdsMuxMatrix/Subsystem  Tag=cdsMuxMatrix  Description=Any size matrix. Inputs and outputs must be connected using Mux and Demux parts.
      settings: AttributesFormatString=%<Tag>
  Mux{1..6} (6 alike) : Mux  Inputs=6
  TM : cdsMuxMatrix/Subsystem  Tag=cdsMuxMatrix  Description=Any size matrix. Inputs and outputs must be connected using Mux and Demux parts.
      settings: AttributesFormatString=%<Tag>
  IPLo : Outport
  IPTo : Outport  Port=2
  IPVo : Outport  Port=3
  IPRo : Outport  Port=4
  IPPo : Outport  Port=5
  IPYo : Outport  Port=6
  BFLo : Outport  Port=7
  BFTo : Outport  Port=8
  BFVo : Outport  Port=9
  BFRo : Outport  Port=10
  BFPo : Outport  Port=11
  BFYo : Outport  Port=12
  MNLo : Outport  Port=13
  MNTo : Outport  Port=14
  MNVo : Outport  Port=15
  MNRo : Outport  Port=16
  MNPo : Outport  Port=17
  MNYo : Outport  Port=18
  IMLo : Outport  Port=19
  IMTo : Outport  Port=20
  IMVo : Outport  Port=21
  IMRo : Outport  Port=22
  IMPo : Outport  Port=23
  IMYo : Outport  Port=24
  TMLo : Outport  Port=25
  TMTo : Outport  Port=26
  TMVo : Outport  Port=27
  TMRo : Outport  Port=28
  TMPop : Outport  Port=29
  TMYo : Outport  Port=30
  MNOLLo : Outport  Port=31
  MNOLTo : Outport  Port=32
  MNOLVo : Outport  Port=33
  MNOLRo : Outport  Port=34
  MNOLPo : Outport  Port=35
  MNOLYo : Outport  Port=36
  wires:
  In6/1 -> Mux2/6
  Mux2/1 -> IP/1
  In3/1 -> Mux2/3
  In1/1 -> Mux2/1
  IP/1 -> Demux3/1
  In5/1 -> Mux2/5
  In2/1 -> Mux2/2
  In4/1 -> Mux2/4
  In12/1 -> Mux1/6
  Mux1/1 -> BF/1
  In9/1 -> Mux1/3
  In7/1 -> Mux1/1
  BF/1 -> Demux1/1
  In11/1 -> Mux1/5
  In8/1 -> Mux1/2
  In10/1 -> Mux1/4
  In18/1 -> Mux3/6
  Mux3/1 -> MN/1
  In15/1 -> Mux3/3
  In13/1 -> Mux3/1
  MN/1 -> Demux2/1
  In17/1 -> Mux3/5
  In14/1 -> Mux3/2
  In16/1 -> Mux3/4
  Mux4/1 -> IM/1
  IM/1 -> Demux4/1
  In30/1 -> Mux4/4
  In27/1 -> Mux4/1
  In29/1 -> Mux4/3
  In28/1 -> Mux4/2
  In32/1 -> Mux4/6
  In31/1 -> Mux4/5
  In38/1 -> Mux5/6
  Mux5/1 -> TM/1
  In35/1 -> Mux5/3
  In33/1 -> Mux5/1
  TM/1 -> Demux5/1
  In37/1 -> Mux5/5
  In34/1 -> Mux5/2
  In36/1 -> Mux5/4
  Demux3/6 -> IPYo/1
  Demux1/1 -> BFLo/1
  Demux1/2 -> BFTo/1
  Demux1/3 -> BFVo/1
  Demux1/4 -> BFRo/1
  Demux1/5 -> BFPo/1
  Demux1/6 -> BFYo/1
  Demux2/1 -> MNLo/1
  Demux2/2 -> MNTo/1
  Demux2/3 -> MNVo/1
  Demux2/4 -> MNRo/1
  Demux2/5 -> MNPo/1
  Demux2/6 -> MNYo/1
  Demux4/1 -> IMLo/1
  Demux4/2 -> IMTo/1
  Demux4/3 -> IMVo/1
  Demux4/4 -> IMRo/1
  Demux4/5 -> IMPo/1
  Demux4/6 -> IMYo/1
  Demux5/1 -> TMLo/1
  Demux3/1 -> IPLo/1
  Demux3/2 -> IPTo/1
  Demux3/3 -> IPVo/1
  Demux3/4 -> IPRo/1
  Demux3/5 -> IPPo/1
  Demux5/2 -> TMTo/1
  Demux5/3 -> TMVo/1
  Demux5/4 -> TMRo/1
  Demux5/5 -> TMPop/1
  Demux5/6 -> TMYo/1
  In24/1 -> Mux6/6
  Mux6/1 -> MNOL/1
  In21/1 -> Mux6/3
  In19/1 -> Mux6/1
  MNOL/1 -> Demux6/1
  In23/1 -> Mux6/5
  In20/1 -> Mux6/2
  In22/1 -> Mux6/4
  Demux6/2 -> MNOLTo/1
  Demux6/3 -> MNOLVo/1
  Demux6/4 -> MNOLRo/1
  Demux6/5 -> MNOLPo/1
  Demux6/6 -> MNOLYo/1
  Demux6/1 -> MNOLLo/1

== system VIS_LIB/MODAL/inputproc_forQUA/EUL ==
  In1 : Inport
  In2 : Inport  Port=2
  In3 : Inport  Port=3
  In4 : Inport  Port=4
  In5 : Inport  Port=5
  In6 : Inport  Port=6
  In7 : Inport  Port=7
  In8 : Inport  Port=8
  In9 : Inport  Port=9
  In10 : Inport  Port=10
  In11 : Inport  Port=11
  In12 : Inport  Port=12
  In13 : Inport  Port=13
  In14 : Inport  Port=14
  In15 : Inport  Port=15
  In16 : Inport  Port=16
  In17 : Inport  Port=17
  In18 : Inport  Port=18
  In19 : Inport  Port=19
  In20 : Inport  Port=20
  In21 : Inport  Port=21
  In22 : Inport  Port=22
  In23 : Inport  Port=23
  In24 : Inport  Port=24
  In25 : Inport  Port=25
  In26 : Inport  Port=26
  In27 : Inport  Port=27
  In28 : Inport  Port=28
  In29 : Inport  Port=29
  In30 : Inport  Port=30
  In31 : Inport  Port=31
  In32 : Inport  Port=32
  In33 : Inport  Port=33
  In34 : Inport  Port=34
  In35 : Inport  Port=35
  In36 : Inport  Port=36
  BF : VIS_LIB/UTILs/FBs_6DOF_DQ
  IM : VIS_LIB/UTILs/FBs_6DOF_DQ
  IP : VIS_LIB/UTILs/FBs_6DOF_DQ
  MN : VIS_LIB/UTILs/FBs_6DOF_DQ
  MNOL : VIS_LIB/UTILs/FBs_6DOF_DQ
  TM : VIS_LIB/UTILs/FBs_6DOF_DQ
  Out1 : Outport
  Out2 : Outport  Port=2
  Out3 : Outport  Port=3
  Out4 : Outport  Port=4
  Out5 : Outport  Port=5
  Out6 : Outport  Port=6
  Out7 : Outport  Port=7
  Out8 : Outport  Port=8
  Out9 : Outport  Port=9
  Out10 : Outport  Port=10
  Out11 : Outport  Port=11
  Out12 : Outport  Port=12
  Out13 : Outport  Port=13
  Out14 : Outport  Port=14
  Out15 : Outport  Port=15
  Out16 : Outport  Port=16
  Out17 : Outport  Port=17
  Out18 : Outport  Port=18
  Out19 : Outport  Port=19
  Out20 : Outport  Port=20
  Out21 : Outport  Port=21
  Out22 : Outport  Port=22
  Out23 : Outport  Port=23
  Out24 : Outport  Port=24
  Out25 : Outport  Port=25
  Out26 : Outport  Port=26
  Out27 : Outport  Port=27
  Out28 : Outport  Port=28
  Out29 : Outport  Port=29
  Out30 : Outport  Port=30
  Out31 : Outport  Port=31
  Out32 : Outport  Port=32
  Out33 : Outport  Port=33
  Out34 : Outport  Port=34
  Out35 : Outport  Port=35
  Out36 : Outport  Port=36
  wires:
  In16/1 -> MN/4
  In15/1 -> MN/3
  In14/1 -> MN/2
  In12/1 -> BF/6
  In13/1 -> MN/1
  In11/1 -> BF/5
  In10/1 -> BF/4
  In9/1 -> BF/3
  In8/1 -> BF/2
  TM/5 -> Out29/1
  TM/2 -> Out26/1
  TM/3 -> Out27/1
  In30/1 -> TM/6
  TM/1 -> Out25/1
  In23/1 -> IM/5
  In22/1 -> IM/4
  In21/1 -> IM/3
  In20/1 -> IM/2
  BF/6 -> Out12/1
  In19/1 -> IM/1
  MN/2 -> Out14/1
  MN/1 -> Out13/1
  In17/1 -> MN/5
  In18/1 -> MN/6
  IM/2 -> Out20/1
  MN/3 -> Out15/1
  IM/1 -> Out19/1
  In24/1 -> IM/6
  TM/4 -> Out28/1
  BF/1 -> Out7/1
  MN/6 -> Out18/1
  MN/5 -> Out17/1
  MN/4 -> Out16/1
  TM/6 -> Out30/1
  In7/1 -> BF/1
  In6/1 -> IP/6
  In5/1 -> IP/5
  In3/1 -> IP/3
  In4/1 -> IP/4
  In29/1 -> TM/5
  In28/1 -> TM/4
  In27/1 -> TM/3
  In26/1 -> TM/2
  BF/5 -> Out11/1
  BF/4 -> Out10/1
  BF/3 -> Out9/1
  BF/2 -> Out8/1
  IP/3 -> Out3/1
  IP/2 -> Out2/1
  IP/1 -> Out1/1
  In1/1 -> IP/1
  In25/1 -> TM/1
  IM/6 -> Out24/1
  IM/5 -> Out23/1
  IM/3 -> Out21/1
  IM/4 -> Out22/1
  In2/1 -> IP/2
  IP/6 -> Out6/1
  IP/5 -> Out5/1
  IP/4 -> Out4/1
  MNOL/5 -> Out35/1
  MNOL/2 -> Out32/1
  MNOL/3 -> Out33/1
  In36/1 -> MNOL/6
  MNOL/4 -> Out34/1
  MNOL/6 -> Out36/1
  In35/1 -> MNOL/5
  In34/1 -> MNOL/4
  In33/1 -> MNOL/3
  In32/1 -> MNOL/2
  In31/1 -> MNOL/1
  MNOL/1 -> Out31/1
